simulink subsystem "P"  (R2024a)
settings: Solver=VariableStepAuto  StartTime=0.0  StopTime=10.0  RelTol=1e-3
undefined symbols (not defined in the file): P_pEnable
settings Model: DefaultTestHarness=P_Harness1  Creator=gordi  LastModifiedBy=gordi

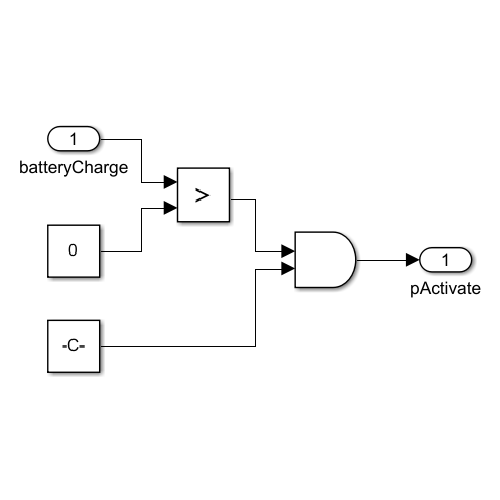
[thumbnail: Simulink's stored preview of the top-level diagram]
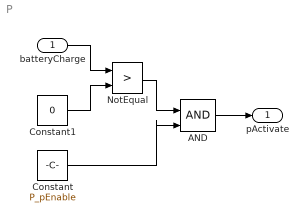
== system P ==
  batteryCharge : Inport
  AND : Logic  IconShape=distinctive  AllPortsSameDT=off  OutDataTypeStr=boolean
  Constant : Constant  Value=P_pEnable
  Constant1 : Constant  Value=0
  NotEqual : RelationalOperator  Operator=>  OutDataTypeStr=boolean  RndMeth=Simplest  InputSameDT=off
  pActivate : Outport
  wires:
  Constant1/1 -> NotEqual/2
  batteryCharge/1 -> NotEqual/1
  NotEqual/1 -> AND/1
  Constant/1 -> AND/2
  AND/1 -> pActivate/1
